simulink model "tugaspsd"  (R2014b)
settings: Solver=ode45  StartTime=0.0  StopTime=10.0  RelTol=1e-3
libraries: simulink x1
settings Model: Creator=User  LastModifiedBy=User

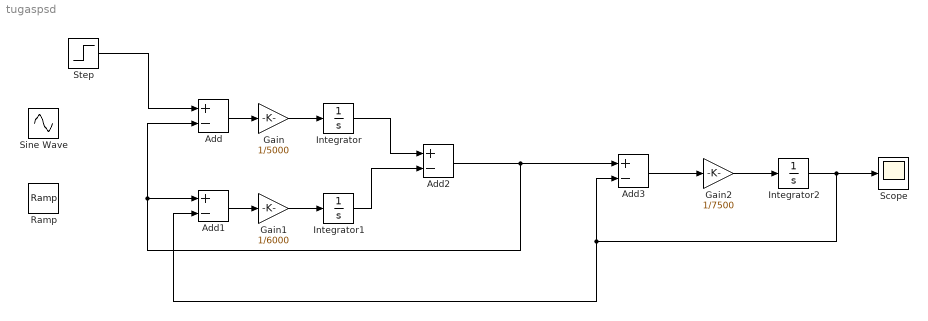
== system tugaspsd ==
  Add{,1..3} (4 alike) : Sum  Inputs=+-
  Gain : Gain  Gain=1/5000
  Gain1 : Gain  Gain=1/6000
  Gain2 : Gain  Gain=1/7500
  Integrator : Integrator
  Integrator1 : Integrator
  Integrator2 : Integrator
  Ramp : simulink/Sources/Ramp  slope=3  start=0  X0=0
  Scope : Scope
      settings: SaveName=tekanan
  Sine Wave : Sin  SampleTime=0
  Step : Step  SampleTime=0
  wires:
  Add/1 -> Gain/1
  Gain/1 -> Integrator/1
  Add1/1 -> Gain1/1
  Gain1/1 -> Integrator1/1
  Add3/1 -> Gain2/1
  Gain2/1 -> Integrator2/1
  Integrator/1 -> Add2/1
  Integrator1/1 -> Add2/2
  Add2/1 -> Add/2, Add1/1, Add3/1
  Integrator2/1 -> Scope/1, Add3/2, Add1/2
  Step/1 -> Add/1
